simulink model "torque_vectoring"  (R2024a)
settings: Solver=VariableStepAuto  StartTime=1026  StopTime=1120  RelTol=1e-3
model workspace (MAT data in the model file):
  SetUp_Conv_Score = Simulink.Parameter
  SetUp_Conv_Score.Complexity = 'real'
  SetUp_Conv_Score.Dimensions = [0 0]
  SetUp_Conv_Score.DataType = 'auto'
undefined symbols (not defined in the file or in its folder): accX, accY, amk_actual_speed, base_torques, dash_se, fl, fr, gyrZ, max_torque_front, max_torque_rear, min_torque_front, min_torque_rear, rl, rr, te_main_APPS, te_main_BPSe, torque_front_n, torque_front_p, torque_rear_n, torque_rear_p, yrc_grip, yrc_ki, yrc_kp_acc, yrc_kp_regen, yrc_ku, yrc_max_power, yrc_steer_factor
libraries: simulink_extras x1, slpidlib x1
settings Model: Creator=andre  LastModifiedBy=britszilla

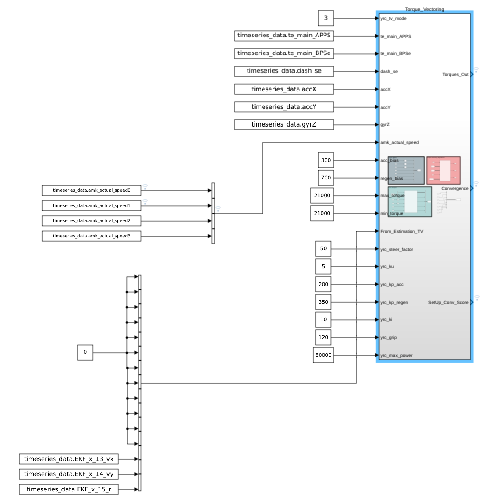
[thumbnail: Simulink's stored preview of the top-level diagram]
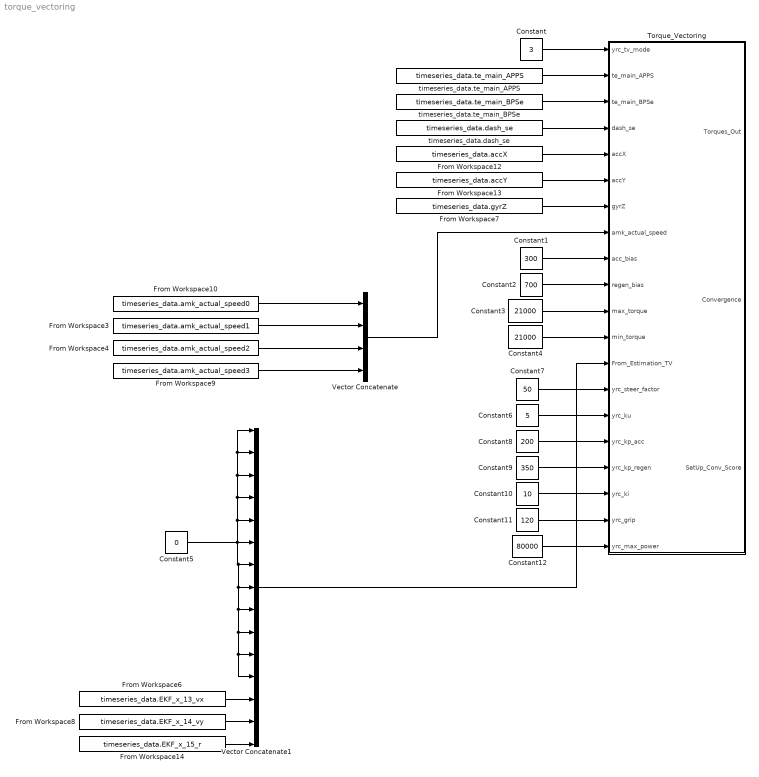
== system torque_vectoring ==
  Constant : Constant  Value=3
  Constant1 : Constant  Value=300
  Constant10 : Constant  Value=10
  Constant11 : Constant  Value=120
  Constant12 : Constant  Value=80000
  Constant2 : Constant  Value=700
  Constant3 : Constant  Value=21000
  Constant4 : Constant  Value=21000
  Constant5 : Constant  Value=0
  Constant6 : Constant  Value=5
  Constant7 : Constant  Value=50
  Constant8 : Constant  Value=200
  Constant9 : Constant  Value=350
  From Workspace10 : FromWorkspace  VariableName=timeseries_data.amk_actual_speed0  OutputAfterFinalValue=Setting to zero
  From Workspace12 : FromWorkspace  VariableName=timeseries_data.accX  OutputAfterFinalValue=Setting to zero
  From Workspace13 : FromWorkspace  VariableName=timeseries_data.accY  OutputAfterFinalValue=Setting to zero
  From Workspace14 : FromWorkspace  VariableName=timeseries_data.EKF_x_15_r  OutputAfterFinalValue=Setting to zero
  From Workspace3 : FromWorkspace  VariableName=timeseries_data.amk_actual_speed1  OutputAfterFinalValue=Setting to zero
  From Workspace4 : FromWorkspace  VariableName=timeseries_data.amk_actual_speed2  OutputAfterFinalValue=Setting to zero
  From Workspace6 : FromWorkspace  VariableName=timeseries_data.EKF_x_13_vx  OutputAfterFinalValue=Setting to zero
  From Workspace7 : FromWorkspace  VariableName=timeseries_data.gyrZ  OutputAfterFinalValue=Setting to zero
  From Workspace8 : FromWorkspace  VariableName=timeseries_data.EKF_x_14_vy  OutputAfterFinalValue=Setting to zero
  From Workspace9 : FromWorkspace  VariableName=timeseries_data.amk_actual_speed3  OutputAfterFinalValue=Setting to zero
  Torque_Vectoring : Subsystem
  Vector Concatenate : Concatenate  NumInputs=4
  Vector Concatenate1 : Concatenate  NumInputs=15
  timeseries_data.dash_se : FromWorkspace  VariableName=timeseries_data.dash_se  OutputAfterFinalValue=Setting to zero
  timeseries_data.te_main_APPS : FromWorkspace  VariableName=timeseries_data.te_main_APPS  OutputAfterFinalValue=Setting to zero
  timeseries_data.te_main_BPSe : FromWorkspace  VariableName=timeseries_data.te_main_BPSe  OutputAfterFinalValue=Setting to zero
  wires:
  Constant/1 -> Torque_Vectoring/1(yrc_tv_mode)
  timeseries_data.te_main_APPS/1 -> Torque_Vectoring/2(te_main_APPS)
  timeseries_data.te_main_BPSe/1 -> Torque_Vectoring/3(te_main_BPSe)
  timeseries_data.dash_se/1 -> Torque_Vectoring/4(dash_se)
  From Workspace12/1 -> Torque_Vectoring/5(accX)
  From Workspace13/1 -> Torque_Vectoring/6(accY)
  From Workspace7/1 -> Torque_Vectoring/7(gyrZ)
  From Workspace10/1 -> Vector Concatenate/1
  From Workspace9/1 -> Vector Concatenate/4
  Vector Concatenate/1 -> Torque_Vectoring/8(amk_actual_speed)
  From Workspace4/1 -> Vector Concatenate/3
  From Workspace3/1 -> Vector Concatenate/2
  Constant1/1 -> Torque_Vectoring/9(acc_bias)
  Constant2/1 -> Torque_Vectoring/10(regen_bias)
  Constant3/1 -> Torque_Vectoring/11(max_torque)
  Constant4/1 -> Torque_Vectoring/12(min_torque)
  From Workspace14/1 -> Vector Concatenate1/15
  From Workspace8/1 -> Vector Concatenate1/14
  From Workspace6/1 -> Vector Concatenate1/13
  Constant5/1 -> Vector Concatenate1/1, Vector Concatenate1/2, Vector Concatenate1/3, Vector Concatenate1/4, Vector Concatenate1/5, Vector Concatenate1/12, Vector Concatenate1/11, Vector Concatenate1/10, Vector Concatenate1/9, Vector Concatenate1/8, Vector Concatenate1/7, Vector Concatenate1/6
  Vector Concatenate1/1 -> Torque_Vectoring/13(From_Estimation_TV)
  Constant7/1 -> Torque_Vectoring/14(yrc_steer_factor)
  Constant6/1 -> Torque_Vectoring/15(yrc_ku)
  Constant8/1 -> Torque_Vectoring/16(yrc_kp_acc)
  Constant9/1 -> Torque_Vectoring/17(yrc_kp_regen)
  Constant10/1 -> Torque_Vectoring/18(yrc_ki)
  Constant11/1 -> Torque_Vectoring/19(yrc_grip)
  Constant12/1 -> Torque_Vectoring/20(yrc_max_power)

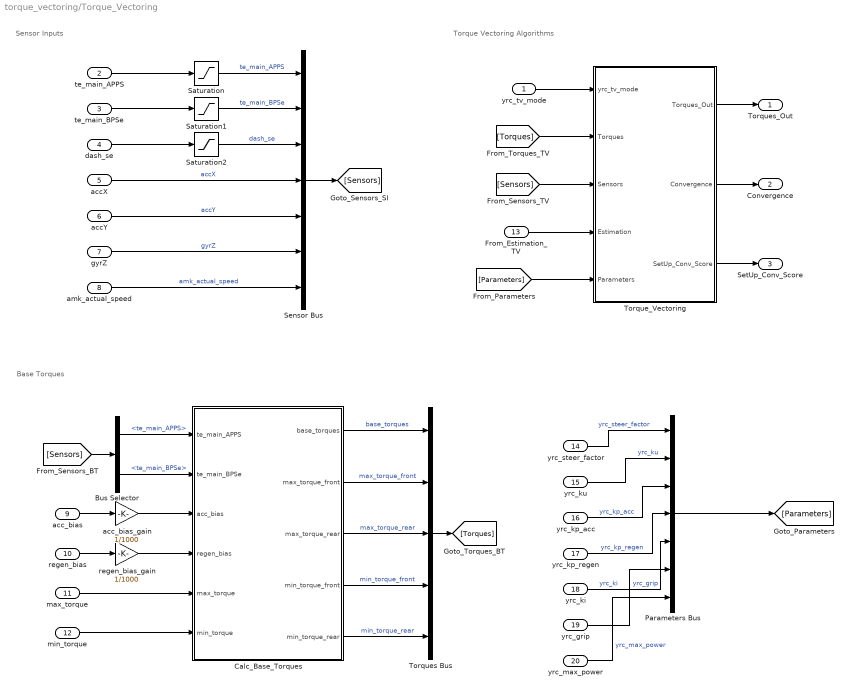
== system torque_vectoring/Torque_Vectoring ==
  note: Sensor Inputs
  note: Base Torques
  note: Torque Vectoring Algorithms
  yrc_tv_mode : Inport
  te_main_APPS : Inport  Port=2
  te_main_BPSe : Inport  Port=3
  dash_se : Inport  Port=4
  accX : Inport  Port=5
  accY : Inport  Port=6
  gyrZ : Inport  Port=7
  amk_actual_speed : Inport  Port=8
  acc_bias : Inport  Port=9
  regen_bias : Inport  Port=10
  max_torque : Inport  Port=11
  min_torque : Inport  Port=12
  From_Estimation_TV : Inport  Port=13
  yrc_steer_factor : Inport  Port=14
  yrc_ku : Inport  Port=15
  yrc_kp_acc : Inport  Port=16
  yrc_kp_regen : Inport  Port=17
  yrc_ki : Inport  Port=18
  yrc_grip : Inport  Port=19
  yrc_max_power : Inport  Port=20
  Bus Selector : BusSelector  OutputSignals=te_main_APPS,te_main_BPSe
  Calc_Base_Torques : Subsystem
  Parameters Bus : BusCreator  Inputs=yrc_steer_factor,yrc_ku,yrc_kp_acc,yrc_kp_regen,yrc_ki,yrc_grip,yrc_max_power
  Saturation : Saturate  UpperLimit=100  LowerLimit=0
  Saturation1 : Saturate  UpperLimit=100  LowerLimit=0
  Saturation2 : Saturate  UpperLimit=127  LowerLimit=-127
  Sensor Bus : BusCreator  Inputs=te_main_APPS,te_main_BPSe,dash_se,accX,accY,gyrZ,amk_actual_speed
  Torque_Vectoring : Subsystem
  Torques Bus : BusCreator  Inputs=base_torques,max_torque_front,max_torque_rear,min_torque_front,min_torque_rear
  acc_bias_gain : Gain  Gain=1/1000
  regen_bias_gain : Gain  Gain=1/1000
  Torques_Out : Outport
  Convergence : Outport  Port=2
  SetUp_Conv_Score : Outport  Port=3
  wires:
  Sensor Bus/1 -> [Sensors]
  te_main_APPS/1 -> Saturation/1
  te_main_BPSe/1 -> Saturation1/1
  dash_se/1 -> Saturation2/1
  accX/1 -> Sensor Bus/4  "accX"
  accY/1 -> Sensor Bus/5  "accY"
  gyrZ/1 -> Sensor Bus/6  "gyrZ"
  amk_actual_speed/1 -> Sensor Bus/7  "amk_actual_speed"
  [Sensors] -> Bus Selector/1
  Saturation/1 -> Sensor Bus/1  "te_main_APPS"
  Saturation1/1 -> Sensor Bus/2  "te_main_BPSe"
  Saturation2/1 -> Sensor Bus/3  "dash_se"
  Bus Selector/1 -> Calc_Base_Torques/1(te_main_APPS)  "<te_main_APPS>"
  Bus Selector/2 -> Calc_Base_Torques/2(te_main_BPSe)  "<te_main_BPSe>"
  acc_bias/1 -> acc_bias_gain/1
  regen_bias/1 -> regen_bias_gain/1
  max_torque/1 -> Calc_Base_Torques/5(max_torque)
  min_torque/1 -> Calc_Base_Torques/6(min_torque)
  acc_bias_gain/1 -> Calc_Base_Torques/3(acc_bias)
  regen_bias_gain/1 -> Calc_Base_Torques/4(regen_bias)
  Calc_Base_Torques/1(base_torques) -> Torques Bus/1  "base_torques"
  Calc_Base_Torques/2(max_torque_front) -> Torques Bus/2  "max_torque_front"
  Calc_Base_Torques/5(min_torque_rear) -> Torques Bus/5  "min_torque_rear"
  Calc_Base_Torques/4(min_torque_front) -> Torques Bus/4  "min_torque_front"
  Calc_Base_Torques/3(max_torque_rear) -> Torques Bus/3  "max_torque_rear"
  Torques Bus/1 -> [Torques]
  yrc_tv_mode/1 -> Torque_Vectoring/1(yrc_tv_mode)
  [Torques] -> Torque_Vectoring/2(Torques)
  [Sensors] -> Torque_Vectoring/3(Sensors)
  Torque_Vectoring/1(Torques_Out) -> Torques_Out/1
  From_Estimation_TV/1 -> Torque_Vectoring/4(Estimation)
  yrc_steer_factor/1 -> Parameters Bus/1  "yrc_steer_factor"
  yrc_ku/1 -> Parameters Bus/2  "yrc_ku"
  Parameters Bus/1 -> [Parameters]
  [Parameters] -> Torque_Vectoring/5(Parameters)
  yrc_kp_acc/1 -> Parameters Bus/3  "yrc_kp_acc"
  yrc_kp_regen/1 -> Parameters Bus/4  "yrc_kp_regen"
  yrc_ki/1 -> Parameters Bus/5  "yrc_ki"
  yrc_grip/1 -> Parameters Bus/6  "yrc_grip"
  yrc_max_power/1 -> Parameters Bus/7  "yrc_max_power"
  Torque_Vectoring/2(Convergence) -> Convergence/1
  Torque_Vectoring/3(SetUp_Conv_Score) -> SetUp_Conv_Score/1

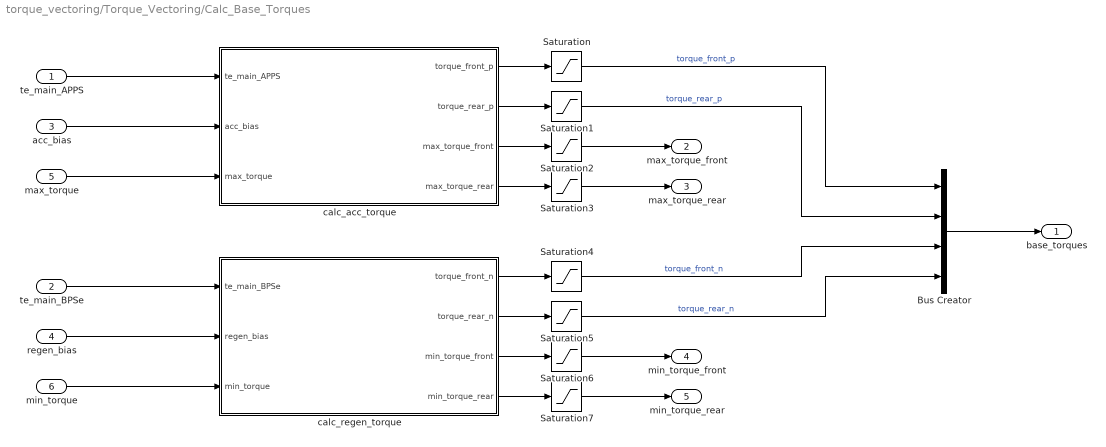
== system torque_vectoring/Torque_Vectoring/Calc_Base_Torques ==
  te_main_APPS : Inport
  te_main_BPSe : Inport  Port=2
  acc_bias : Inport  Port=3
  regen_bias : Inport  Port=4
  max_torque : Inport  Port=5
  min_torque : Inport  Port=6
  Bus Creator : BusCreator  Inputs=torque_front_p,torque_rear_p,torque_front_n,torque_rear_n
  Saturation{,1..3} (4 alike) : Saturate  UpperLimit=21000  LowerLimit=0
  Saturation{4..7} (4 alike) : Saturate  UpperLimit=0  LowerLimit=-21000
  calc_acc_torque : MATLAB Function  TreatAsAtomicUnit=on
  calc_regen_torque : MATLAB Function  TreatAsAtomicUnit=on
  base_torques : Outport
  max_torque_front : Outport  Port=2
  max_torque_rear : Outport  Port=3
  min_torque_front : Outport  Port=4
  min_torque_rear : Outport  Port=5
  wires:
  te_main_APPS/1 -> calc_acc_torque/1(te_main_APPS)
  acc_bias/1 -> calc_acc_torque/2(acc_bias)
  max_torque/1 -> calc_acc_torque/3(max_torque)
  te_main_BPSe/1 -> calc_regen_torque/1(te_main_BPSe)
  regen_bias/1 -> calc_regen_torque/2(regen_bias)
  min_torque/1 -> calc_regen_torque/3(min_torque)
  calc_acc_torque/1(torque_front_p) -> Saturation/1
  calc_acc_torque/2(torque_rear_p) -> Saturation1/1
  calc_acc_torque/3(max_torque_front) -> Saturation2/1
  calc_acc_torque/4(max_torque_rear) -> Saturation3/1
  calc_regen_torque/1(torque_front_n) -> Saturation4/1
  calc_regen_torque/2(torque_rear_n) -> Saturation5/1
  calc_regen_torque/3(min_torque_front) -> Saturation6/1
  calc_regen_torque/4(min_torque_rear) -> Saturation7/1
  Saturation2/1 -> max_torque_front/1
  Saturation3/1 -> max_torque_rear/1
  Saturation6/1 -> min_torque_front/1
  Saturation7/1 -> min_torque_rear/1
  Bus Creator/1 -> base_torques/1
  Saturation/1 -> Bus Creator/1  "torque_front_p"
  Saturation1/1 -> Bus Creator/2  "torque_rear_p"
  Saturation4/1 -> Bus Creator/3  "torque_front_n"
  Saturation5/1 -> Bus Creator/4  "torque_rear_n"

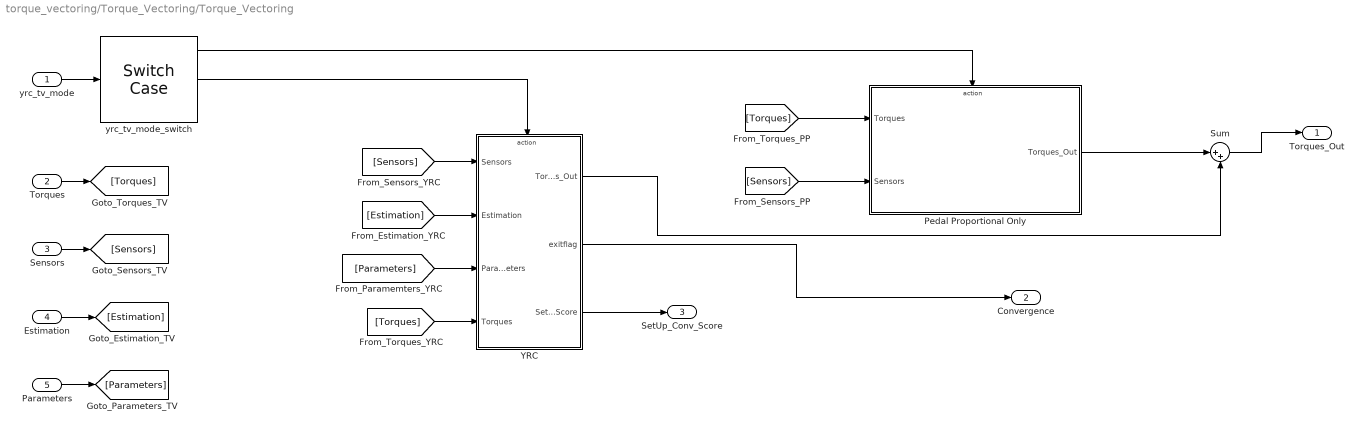
== system torque_vectoring/Torque_Vectoring/Torque_Vectoring ==
  yrc_tv_mode : Inport
  Torques : Inport  Port=2
  Sensors : Inport  Port=3
  Estimation : Inport  Port=4
  Parameters : Inport  Port=5
  Pedal Proportional Only : Subsystem
  Sum : Sum  Inputs=|++
  YRC : Subsystem
  yrc_tv_mode_switch : SwitchCase  CaseConditions={1,3}
  Torques_Out : Outport
  Convergence : Outport  Port=2
  SetUp_Conv_Score : Outport  Port=3
  wires:
  Torques/1 -> [Torques]
  Sensors/1 -> [Sensors]
  yrc_tv_mode/1 -> yrc_tv_mode_switch/1
  [Torques] -> Pedal Proportional Only/1(Torques)
  yrc_tv_mode_switch/1 -> Pedal Proportional Only/Action
  [Sensors] -> Pedal Proportional Only/2(Sensors)
  yrc_tv_mode_switch/2 -> YRC/Action
  [Sensors] -> YRC/1(Sensors)
  Estimation/1 -> [Estimation]
  [Estimation] -> YRC/2(Estimation)
  Parameters/1 -> [Parameters]
  [Parameters] -> YRC/3(Parameters)
  [Torques] -> YRC/4(Torques)
  YRC/1(Torques_Out) -> Sum/2
  Pedal Proportional Only/1(Torques_Out) -> Sum/1
  Sum/1 -> Torques_Out/1
  YRC/2(exitflag) -> Convergence/1
  YRC/3(SetUp_Conv_Score) -> SetUp_Conv_Score/1

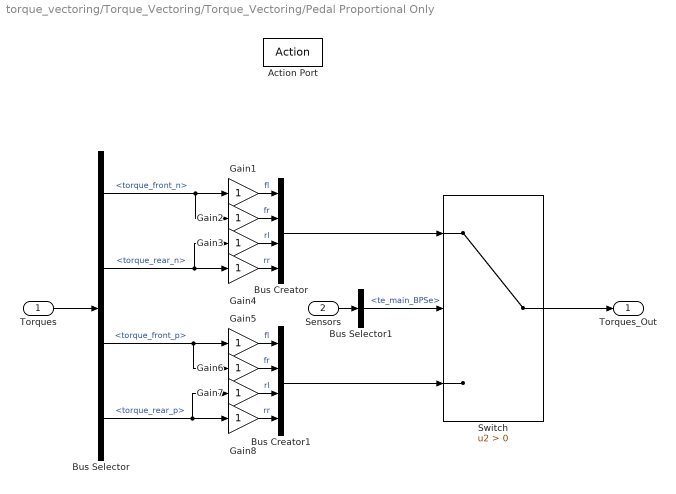
== system torque_vectoring/Torque_Vectoring/Torque_Vectoring/Pedal Proportional Only ==
  Torques : Inport
  Sensors : Inport  Port=2
  Action Port : ActionPort  ActionPortLabel=case [ 1 ]:
  Bus Creator : BusCreator  Inputs=fl,fr,rl,rr
  Bus Creator1 : BusCreator  Inputs=fl,fr,rl,rr
  Bus Selector : BusSelector  OutputSignals=base_torques.torque_front_n,base_torques.torque_rear_n,base_torques.torque_front_p,base_torques.torque_rear_p
  Bus Selector1 : BusSelector  OutputSignals=te_main_BPSe
  Gain{1..3,5..8} (7 alike) : Gain
  Gain4 : Gain  RndMeth=Zero
  Switch : Switch  Criteria=u2 > Threshold  SaturateOnIntegerOverflow=off  InputSameDT=off
  Torques_Out : Outport
  wires:
  Torques/1 -> Bus Selector/1
  Sensors/1 -> Bus Selector1/1
  Switch/1 -> Torques_Out/1
  Bus Selector1/1 -> Switch/2  "<te_main_BPSe>"
  Gain1/1 -> Bus Creator/1  "fl"
  Gain2/1 -> Bus Creator/2  "fr"
  Gain3/1 -> Bus Creator/3  "rl"
  Gain4/1 -> Bus Creator/4  "rr"
  Gain5/1 -> Bus Creator1/1  "fl"
  Gain6/1 -> Bus Creator1/2  "fr"
  Gain7/1 -> Bus Creator1/3  "rl"
  Gain8/1 -> Bus Creator1/4  "rr"
  Bus Selector/1 -> Gain2/1, Gain1/1  "<torque_front_n>"
  Bus Selector/2 -> Gain3/1, Gain4/1  "<torque_rear_n>"
  Bus Selector/3 -> Gain6/1, Gain5/1  "<torque_front_p>"
  Bus Selector/4 -> Gain7/1, Gain8/1  "<torque_rear_p>"
  Bus Creator/1 -> Switch/1
  Bus Creator1/1 -> Switch/3

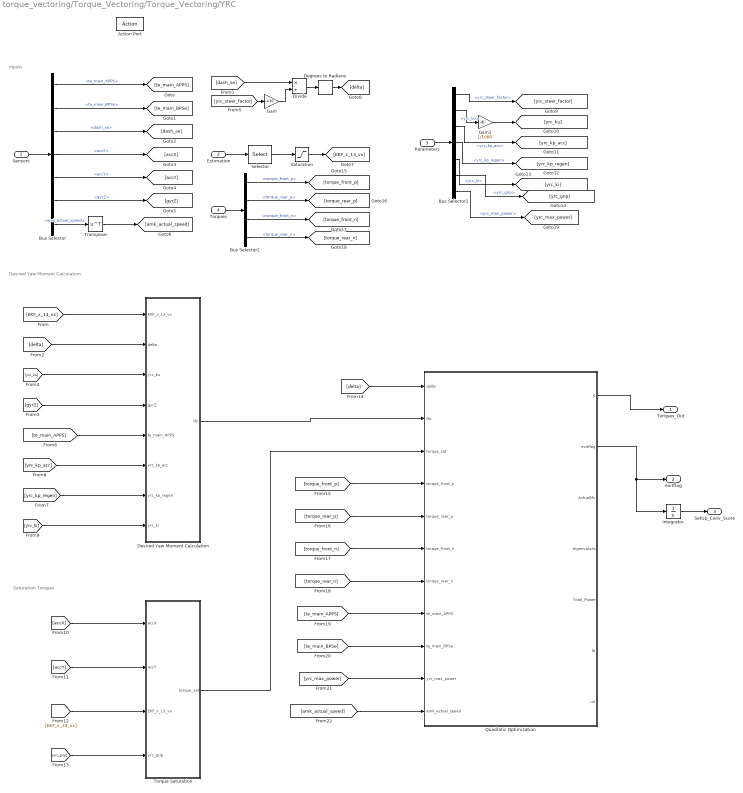
== system torque_vectoring/Torque_Vectoring/Torque_Vectoring/YRC ==
  note: Inputs
  note: Desired Yaw Moment Calculation
  note: Saturation Torques
  Sensors : Inport
  Estimation : Inport  Port=2
  Parameters : Inport  Port=3
  Torques : Inport  Port=4
  Action Port : ActionPort  ActionPortLabel=case [ 3 ]:
  Bus Selector : BusSelector  OutputSignals=te_main_APPS,te_main_BPSe,dash_se,accX,accY,gyrZ,amk_actual_speed
  Bus Selector1 : BusSelector  OutputSignals=yrc_steer_factor,yrc_ku,yrc_kp_acc,yrc_kp_regen,yrc_ki,yrc_grip,yrc_max_power
  Bus Selector2 : BusSelector  OutputSignals=base_torques.torque_front_p,base_torques.torque_rear_p,base_torques.torque_front_n,base_torques.torque_rear_n
  Degrees to Radians : simulink_extras/Transformations/Degrees to Radians
  Desired Yaw Moment Calculation : Subsystem
  Divide : Product  Inputs=*/
  Gain : Gain  Gain=-1/10
  Gain1 : Gain  Gain=1/1000
  Integrator : Integrator
  Quadratic Optimization : MATLAB Function  TreatAsAtomicUnit=on
  Saturation : Saturate  UpperLimit=35  LowerLimit=0
  Selector : Selector  InputPortWidth=15  IndexOptions=Index vector (dialog)  Indices=[13]  OutputSizes=1
  Torque Saturation : Subsystem
  Transpose : Math  Operator=transpose
  Torques_Out : Outport
  exitflag : Outport  Port=2
  SetUp_Conv_Score : Outport  Port=3
  wires:
  Sensors/1 -> Bus Selector/1
  Bus Selector/1 -> [te_main_APPS]  "<te_main_APPS>"
  Bus Selector/2 -> [te_main_BPSe]  "<te_main_BPSe>"
  Bus Selector/3 -> [dash_se]  "<dash_se>"
  Bus Selector/4 -> [accX]  "<accX>"
  Bus Selector/5 -> [accY]  "<accY>"
  Bus Selector/6 -> [gyrZ]  "<gyrZ>"
  Bus Selector/7 -> Transpose/1  "<amk_actual_speed>"
  Estimation/1 -> Selector/1
  Selector/1 -> Saturation/1
  Saturation/1 -> [EKF_x_13_vx]
  [EKF_x_13_vx] -> Desired Yaw Moment Calculation/1(EKF_x_13_vx)
  [dash_se] -> Divide/1
  [delta] -> Desired Yaw Moment Calculation/2(delta)
  Parameters/1 -> Bus Selector1/1
  Bus Selector1/1 -> [yrc_steer_factor]  "<yrc_steer_factor>"
  [yrc_ku] -> Desired Yaw Moment Calculation/3(yrc_ku)
  Bus Selector1/2 -> Gain1/1  "<yrc_ku>"
  Gain1/1 -> [yrc_ku]
  [yrc_steer_factor] -> Gain/1
  Gain/1 -> Divide/2
  Divide/1 -> Degrees to Radians/1
  Degrees to Radians/1 -> [delta]
  [gyrZ] -> Desired Yaw Moment Calculation/4(gyrZ)
  [te_main_APPS] -> Desired Yaw Moment Calculation/5(te_main_APPS)
  Bus Selector1/3 -> [yrc_kp_acc]  "<yrc_kp_acc>"
  Bus Selector1/4 -> [yrc_kp_regen]  "<yrc_kp_regen>"
  [yrc_kp_acc] -> Desired Yaw Moment Calculation/6(yrc_kp_acc)
  [yrc_kp_regen] -> Desired Yaw Moment Calculation/7(yrc_kp_regen)
  Bus Selector1/5 -> [yrc_ki]  "<yrc_ki>"
  [yrc_ki] -> Desired Yaw Moment Calculation/8(yrc_ki)
  [accY] -> Torque Saturation/2(accY)
  [accX] -> Torque Saturation/1(accX)
  [EKF_x_13_vx] -> Torque Saturation/3(EKF_x_13_vx)
  [yrc_grip] -> Torque Saturation/4(yrc_grip)
  Bus Selector1/6 -> [yrc_grip]  "<yrc_grip>"
  [delta] -> Quadratic Optimization/1(delta)
  Desired Yaw Moment Calculation/1(Mz) -> Quadratic Optimization/2(Mz)
  Torque Saturation/1(torque_sat) -> Quadratic Optimization/3(torque_sat)
  Torques/1 -> Bus Selector2/1
  Bus Selector2/1 -> [torque_front_p]  "<torque_front_p>"
  Bus Selector2/4 -> [torque_rear_n]  "<torque_rear_n>"
  Bus Selector2/3 -> [torque_front_n]  "<torque_front_n>"
  Bus Selector2/2 -> [torque_rear_p]  "<torque_rear_p>"
  [torque_front_p] -> Quadratic Optimization/4(torque_front_p)
  [torque_rear_p] -> Quadratic Optimization/5(torque_rear_p)
  [torque_front_n] -> Quadratic Optimization/6(torque_front_n)
  [torque_rear_n] -> Quadratic Optimization/7(torque_rear_n)
  [te_main_APPS] -> Quadratic Optimization/8(te_main_APPS)
  [te_main_BPSe] -> Quadratic Optimization/9(te_main_BPSe)
  Bus Selector1/7 -> [yrc_max_power]  "<yrc_max_power>"
  [yrc_max_power] -> Quadratic Optimization/10(yrc_max_power)
  [amk_actual_speed] -> Quadratic Optimization/11(amk_actual_speed)
  Transpose/1 -> [amk_actual_speed]
  Quadratic Optimization/1(X) -> Torques_Out/1
  Quadratic Optimization/2(exitflag) -> Integrator/1, exitflag/1
  Integrator/1 -> SetUp_Conv_Score/1

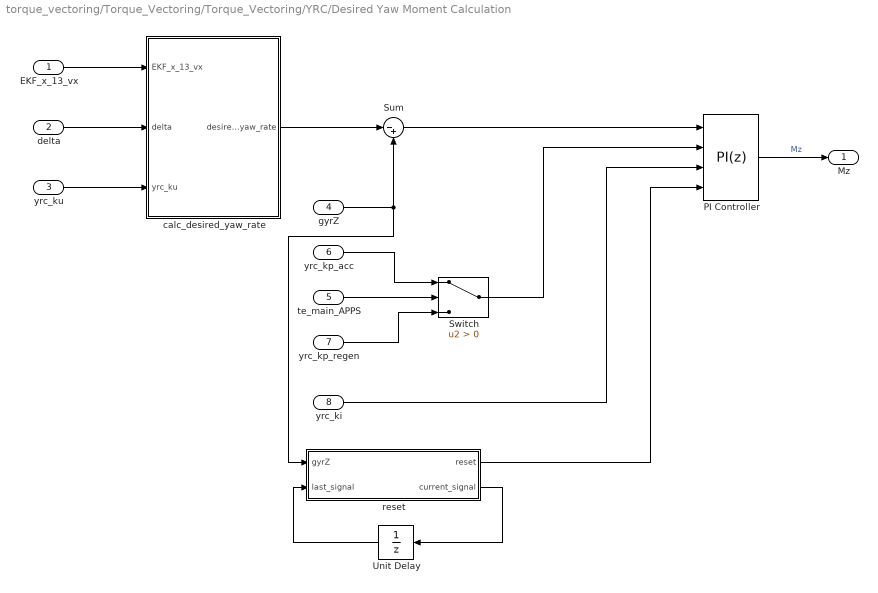
== system torque_vectoring/Torque_Vectoring/Torque_Vectoring/YRC/Desired Yaw Moment Calculation ==
  EKF_x_13_vx : Inport
  delta : Inport  Port=2
  yrc_ku : Inport  Port=3
  gyrZ : Inport  Port=4
  te_main_APPS : Inport  Port=5
  yrc_kp_acc : Inport  Port=6
  yrc_kp_regen : Inport  Port=7
  yrc_ki : Inport  Port=8
  PI Controller : slpidlib/PID Controller  Controller=PI  Form=Parallel  TimeDomain=Discrete-time  UseExternalTs=off  SampleTime=-1  IntegratorMethod=Backward Euler  FilterMethod=Forward Euler  ControllerParametersSource=external  P=400  I=100  UseKiTs=off  D=10  UseExternalDerivativeSource=off  N=1  UseFilter=on  TunerSelectOption=Transfer Function Based (PID Tuner App)  InitialConditionSource=internal  InitialConditionForIntegrator=0  InitialConditionForFilter=0  DifferentiatorICPrevScaledInput=0  ExternalReset=rising  TrackingMode=off  Kt=1  LimitOutput=on  SatLimitsSource=internal  UpperSaturationLimit=1700  LowerSaturationLimit=-1700  LinearizeAsGain=off  AntiWindupMode=clamping  Kb=6  LimitIntegrator=off  UpperIntegratorSaturationLimit=inf  LowerIntegratorSaturationLimit=-inf  POutMin=[]  POutMax=[]  IOutMin=[]  IOutMax=[]  DOutMin=[]  DOutMax=[]  NOutMin=[]  NOutMax=[]  SumOutMin=[]  SumOutMax=[]  SaturationOutMin=[]  SaturationOutMax=[]  PParamMin=[]  PParamMax=[]  IParamMin=[]  IParamMax=[]  DParamMin=[]  DParamMax=[]  NParamMin=[]  NParamMax=[]  KbParamMin=[]  KbParamMax=[]  KtParamMin=[]  KtParamMax=[]  KbOutMin=[]  KbOutMax=[]  KtOutMin=[]  KtOutMax=[]  IntegratorOutMin=[]  IntegratorOutMax=[]  FilterOutMin=[]  FilterOutMax=[]  SumI1OutMin=[]  SumI1OutMax=[]  SumI2OutMin=[]  SumI2OutMax=[]  SumI3OutMin=[]  SumI3OutMax=[]  SumI4OutMin=[]  SumI4OutMax=[]  SumDOutMin=[]  SumDOutMax=[]  DifferentiatorOutMin=[]  DifferentiatorOutMax=[]  FilterDiffOutCoefMin=[]  FilterDiffOutCoefMax=[]  ReciprocalOutMin=[]  ReciprocalOutMax=[]  SumDenOutMin=[]  SumDenOutMax=[]  SumNumOutMin=[]  SumNumOutMax=[]  DivideOutMin=[]  DivideOutMax=[]  UdiffTsProdOutMin=[]  UdiffTsProdOutMax=[]  NTsProdOutMin=[]  NTsProdOutMax=[]  UintegralTsProdOutMin=[]  UintegralTsProdOutMax=[]  UngainTsProdOutMin=[]  UngainTsProdOutMax=[]  ClampingZeroOutDataTypeStr=Inherit: Inherit via back propagation  ClampingZeroOutMin=[]  ClampingZeroOutMax=[]  FilterDenConstantOutDataTypeStr=Inherit: Inherit via back propagation  FilterDenConstantOutMin=[]  FilterDenConstantOutMax=[]  PCopyOutDataTypeStr=Inherit: Inherit via back propagation  PCopyOutMin=[]  PCopyOutMax=[]  NCopyOutDataTypeStr=Inherit: Inherit via back propagation  NCopyOutMin=[]  NCopyOutMax=[]  IntegratorContinuousStateAttributes=''  IntegratorStateMustResolveToSignalObject=off  IntegratorRTWStateStorageClass=Auto  FilterContinuousStateAttributes=''  FilterStateMustResolveToSignalObject=off  FilterRTWStateStorageClass=Auto  ParallelPVariant=ExternalParameters  IdealPVariant=Disabled  IVariant=ExternalParameters  DVariant=Disabled  IntegratorVariant=Discrete  SatVariant=Enabled  AWVariant=DiscClampingParallel  PCopyVariant=Disabled  TRVariant=Disabled  FdbkBlocksVariant=Feedback  IdealPFdbkVariant=Passthrough  SatFdbkVariant=Passthrough  DerivativeFilterVariant=Disabled  NVariant=Disabled  NCopyVariant=Disabled_SignalSpec  FilterICVariant=Disabled  IntegratorICVariant=InternalICs  ExternalResetVariant=ExternalReset  TRSumVariant=Passthrough  SumFdbkVariant=Enabled  SumVariant=Sum_PI  TsampFilterVariant=InternalTs  TsampNgainVariant=Passthrough  TsampIntegralVariant=Disabled_SignalSpec  ExternalSaturationOutDataTypeStr=Inherit: Same as second input  DerivativeSourceVariant=Disabled
  Sum : Sum  Inputs=|-+
  Switch : Switch  Criteria=u2 > Threshold  SaturateOnIntegerOverflow=off  InputSameDT=off
  Unit Delay : UnitDelay  SampleTime=-1  HasFrameUpgradeWarning=on
  calc_desired_yaw_rate : MATLAB Function  TreatAsAtomicUnit=on
  reset : MATLAB Function  TreatAsAtomicUnit=on
  Mz : Outport
  wires:
  EKF_x_13_vx/1 -> calc_desired_yaw_rate/1(EKF_x_13_vx)
  delta/1 -> calc_desired_yaw_rate/2(delta)
  yrc_ku/1 -> calc_desired_yaw_rate/3(yrc_ku)
  calc_desired_yaw_rate/1(desired_yaw_rate) -> Sum/1
  gyrZ/1 -> reset/1(gyrZ), Sum/2
  Sum/1 -> PI Controller/1
  te_main_APPS/1 -> Switch/2
  yrc_kp_acc/1 -> Switch/1
  yrc_kp_regen/1 -> Switch/3
  Switch/1 -> PI Controller/2
  yrc_ki/1 -> PI Controller/3
  reset/2(current_signal) -> Unit Delay/1
  Unit Delay/1 -> reset/2(last_signal)
  reset/1(reset) -> PI Controller/4
  PI Controller/1 -> Mz/1  "Mz"

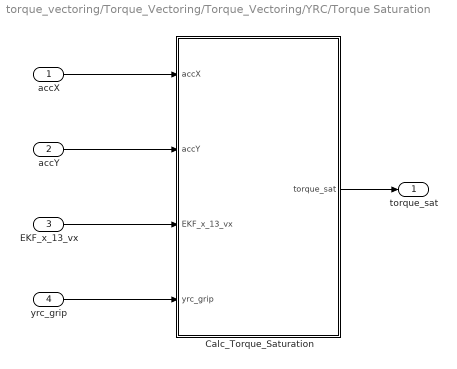
== system torque_vectoring/Torque_Vectoring/Torque_Vectoring/YRC/Torque Saturation ==
  accX : Inport
  accY : Inport  Port=2
  EKF_x_13_vx : Inport  Port=3
  yrc_grip : Inport  Port=4
  Calc_Torque_Saturation : MATLAB Function  TreatAsAtomicUnit=on
  torque_sat : Outport
  wires:
  accX/1 -> Calc_Torque_Saturation/1(accX)
  accY/1 -> Calc_Torque_Saturation/2(accY)
  EKF_x_13_vx/1 -> Calc_Torque_Saturation/3(EKF_x_13_vx)
  yrc_grip/1 -> Calc_Torque_Saturation/4(yrc_grip)
  Calc_Torque_Saturation/1(torque_sat) -> torque_sat/1

== matlab function torque_vectoring/Torque_Vectoring/Calc_Base_Torques/calc_regen_torque ==
  data: te_main_BPSe input; torque_front_n output; regen_bias input; min_torque input; torque_rear_n output; min_torque_front output; min_torque_rear output
function [torque_front_n, torque_rear_n, min_torque_front, min_torque_rear] = ...
    calc_regen_torque(te_main_BPSe, regen_bias, min_torque)

if regen_bias > 0.5
    min_torque_front = - min_torque;
    min_torque_rear = - (min_torque * (1 - regen_bias)) / regen_bias;
else
    min_torque_front = - (min_torque * regen_bias) / (1 - regen_bias);
    min_torque_rear = - min_torque;
end

if te_main_BPSe > 0
    torque_front_n = min_torque_front * (te_main_BPSe / 100);
    torque_rear_n = min_torque_rear * (te_main_BPSe / 100);
else
    torque_front_n = 0;
    torque_rear_n = 0;
end

end

== matlab function torque_vectoring/Torque_Vectoring/Calc_Base_Torques/calc_acc_torque ==
  data: te_main_APPS input; torque_front_p output; acc_bias input; max_torque input; torque_rear_p output; max_torque_front output; max_torque_rear output
function [torque_front_p, torque_rear_p, max_torque_front, max_torque_rear] = ...
    calc_acc_torque(te_main_APPS, acc_bias, max_torque)

if acc_bias > 0.5
    max_torque_front = max_torque;
    max_torque_rear = (max_torque * (1 - acc_bias)) / acc_bias;
else
    max_torque_front = (max_torque * acc_bias) / (1 - acc_bias);
    max_torque_rear = max_torque;
end

if te_main_APPS > 0
    torque_front_p = max_torque_front * (te_main_APPS / 100);
    torque_rear_p = max_torque_rear * (te_main_APPS / 100);
else
    torque_front_p = 0;
    torque_rear_p = 0;
end

end

== matlab function torque_vectoring/Torque_Vectoring/Torque_Vectoring/YRC/Desired Yaw Moment Calculation/calc_desired_yaw_rate ==
  data: EKF_x_13_vx input; desired_yaw_rate output; delta input; yrc_ku input
function desired_yaw_rate = calc_desired_yaw_rate(EKF_x_13_vx, delta, yrc_ku)

wheelbase = 1.54;
desired_yaw_rate = (EKF_x_13_vx * delta) / (wheelbase + yrc_ku*EKF_x_13_vx^2);

== matlab function torque_vectoring/Torque_Vectoring/Torque_Vectoring/YRC/Desired Yaw Moment Calculation/reset ==
  data: gyrZ input; reset output; last_signal input; current_signal output
function [reset, current_signal] = reset(gyrZ, last_signal)

if last_signal == sign(gyrZ)
    reset = 0;
else
    reset = 1;
end
current_signal = sign(gyrZ);
end

== matlab function torque_vectoring/Torque_Vectoring/Torque_Vectoring/YRC/Torque Saturation/Calc_Torque_Saturation ==
  data: accX input; torque_sat output; accY input; EKF_x_13_vx input; yrc_grip input
function torque_sat = calc_torque_saturation(accX, accY, EKF_x_13_vx, yrc_grip)

mass = 302;
wheelbase = 1.54;
track_front = 1.2;
track_rear = 1.2;
height_cg = 0.331;
weight_dist = 0.48;
g = 9.81;
area = 1;
CL = 4.64;
rho = 1.23;
aero_dist = 0.48;
r = 0.235;
GR = 15.21;
mu_x = yrc_grip / 100;
slope_mu = 0.00035;

stationary_front = weight_dist*mass*g;
stationary_rear = (1-weight_dist)*mass*g;

lateral_front = (mass*height_cg*accY)/track_front;
lateral_rear = (mass*height_cg*accY)/track_rear;

longitudinal = (mass*height_cg*accX)/wheelbase;

CL_front = CL*aero_dist;
CL_rear = CL*(1-aero_dist);

lift_front = 0.5*CL_front*rho*EKF_x_13_vx^2*area;
lift_rear = 0.5*CL_rear*rho*EKF_x_13_vx^2*area;

Fz = zeros(4,1);

Fz(1) = stationary_front/2 - longitudinal/2 - lateral_front/2 + lift_front/2;
Fz(2) = stationary_front/2 - longitudinal/2 + lateral_front/2 + lift_front/2;
Fz(3) = stationary_rear/2  + longitudinal/2 - lateral_rear/2  + lift_rear/2;
Fz(4) = stationary_rear/2  + longitudinal/2 + lateral_rear/2  + lift_rear/2;

torque_sat = zeros(4,1);

torque_sat(1) = (Fz(1) * max(mu_x - slope_mu * Fz(1), 1)) / GR * r * 1000;
torque_sat(2) = (Fz(2) * max(mu_x - slope_mu * Fz(2), 1)) / GR * r * 1000;
torque_sat(3) = (Fz(3) * max(mu_x - slope_mu * Fz(3), 1)) / GR * r * 1000;
torque_sat(4) = (Fz(4) * max(mu_x - slope_mu * Fz(4), 1)) / GR * r * 1000;

end

== matlab function torque_vectoring/Torque_Vectoring/Torque_Vectoring/YRC/Quadratic Optimization ==
  data: delta input; Mz input; torque_sat input; torque_front_p input; X output; exitflag output; ActualMz output; eigenvalues output; Total_Power output; torque_rear_p input; torque_front_n input; torque_rear_n input; te_main_APPS input; te_main_BPSe input; lb output; ub output; yrc_max_power input; amk_actual_speed input
function [X, exitflag, ActualMz, eigenvalues, Total_Power, lb, ub] = quadratic_optimization(delta, Mz, torque_sat,...
    torque_front_p, torque_rear_p, torque_front_n, torque_rear_n,...
    te_main_APPS, te_main_BPSe, yrc_max_power, amk_actual_speed)

t = 1.2;
wr = 0.235;
a = 0.74;
GR = 15.21;

K = zeros(4,1);
K(1) = (GR / wr) * ((-cos(delta) * t) / 2 + sin(delta) * a);
K(2) = (GR / wr) * (( cos(delta) * t) / 2 + sin(delta) * a);
K(3) = (GR / wr) * (-t / 2);
K(4) = (GR / wr) * ( t / 2);

H1 = K*K';
f = -2*Mz*K;

H2 = diag([1/torque_sat(1)^2, 1/torque_sat(2)^2, 1/torque_sat(3)^2, 1/torque_sat(4)^2]);

lambda1 = 1;
lambda2 = 2;
lambda3 = 0;


%Total H Matrix

H = lambda1*H1 + lambda2*H2 + lambda3*eye(4);
eigenvalues = eig(H);

%% Constraints


lb = [max(torque_front_n, -torque_sat(1)),...
      max(torque_front_n, -torque_sat(2)),...
      max(torque_rear_n,  -torque_sat(3)),...
      max(torque_rear_n,  -torque_sat(4))];

if te_main_APPS >= 0 %Acceleration
    
    ub = [min(torque_front_p, torque_sat(1)),...
          min(torque_front_p, torque_sat(2)),...
          min(torque_rear_p, torque_sat(3)),...
          min(torque_rear_p, torque_sat(4))];

    [torque_requested] = torque_requested_acc(amk_actual_speed, yrc_max_power, ub);

    b_eq = torque_requested * te_main_APPS / 100;

    X0 = ub.*te_main_APPS/100;

else  %Braking

    ub = [0, 0, 0, 0];
  
    [torque_requested] = torque_requested_regen(amk_actual_speed, yrc_max_power, lb);

    b_eq = torque_requested * te_main_BPSe / 100;

    X0 = lb.*te_main_BPSe/100;

end

%Equality Constraint, b_eq already defined
A_eq = [1, 1, 1, 1];


%Inequality Constraints, cap by power

if te_main_APPS >= 0 % Acceleration
    A = amk_actual_speed;
    b = yrc_max_power;


else % Regen, Negative Torque requires Negative sign to achieve A*x <= b form with max power
    A = - amk_actual_speed;
    b = yrc_max_power;

end


%% Solve

options = optimoptions('quadprog','Algorithm','active-set','Display','off','MaxIterations',500);

%disp(te_main_APPS)
%disp(b_eq)

[X, ~, exitflag] = quadprog(H, f, A, b, A_eq, b_eq, lb, ub, X0, options);

if exitflag == 1
disp("X =");
disp(X);
end


Total_Power = dot(amk_actual_speed, X);

ActualMz = dot(K, X);

end


%% Utilities

function [torque_requested] = torque_requested_acc(amk_actual_speed, yrc_max_power, ub)

    %[~, sorted_idx] = sort(amk_actual_speed); This changes wheel order
    P = zeros(1,4);
    T = zeros(1,4);
    for i = 1:length(amk_actual_speed)
        P(i) = amk_actual_speed(i).*ub(i);
        T(i) = ub(i);
        if sum(P) > yrc_max_power
            T(i) = (yrc_max_power - (sum(P) - P(i))) ./ amk_actual_speed(i);
        end
    end
    torque_requested = sum(T);
end

function [torque_requested] = torque_requested_regen(amk_actual_speed, yrc_max_power, lb)

    %[~, sorted_idx] = sort(amk_actual_speed); This changes wheel order
    P = zeros(1,4);
    T = zeros(1,4);
    for i = 1:length(amk_actual_speed)
        P(i) = amk_actual_speed(i).*lb(i);
        T(i) = lb(i);
        if sum(P) < yrc_max_power
            T(i) = (yrc_max_power - (sum(P) - P(i))) ./ amk_actual_speed(i);
        end
    end
    torque_requested = sum(T);
end
